simulink model "line_fit"  (Simulink 8.4)
settings: Solver=FixedStepDiscrete  SolverMode=SingleTasking  StartTime=0.0  StopTime=inf  RelTol=1e-3
model workspace (MATLAB code in the model file):
  | FracPeriod=0.5; % fraction of period of sinusoid that we will match
  | N=56; %Total number points for estimate
  | Npoly=2; % Order of polynomial to use in fitting
  | Duration = 2; % Total length of observation window
  | Ts = Duration / N; % Sample interval
undefined symbols (not defined in the file): NN
libraries: dspstat3 x3, dspsrcs4 x2, simulink x2, dsppolyfun x1, dspsnks4 x1
CloseFcn:
  | clear FixPtSimRanges;
settings Model: DataTypeOverride=Double  MinMaxOverflowLogging=MinMaxAndOverflow  Creator=Dick Benson  LastModifiedBy=Dick  ExtModeAutoUpdateStatusClock=off
settings DataIOCC: SaveOutput=off  SignalLogging=off  SaveTime=off
settings OptimizationCC: InlineParams=on  InitFltsAndDblsToZero=on
settings DebuggingCC: SignalResolutionControl=TryResolveAllWithWarning  SolverPrmCheckMsg=none
settings HardwareCC: ProdHWDeviceType=ASIC/FPGA  TargetLongLongMode=on  TargetEndianess=LittleEndian  TargetHWDeviceType=MATLAB Host  ProdEqTarget=off
settings SFSimCC: SimParseCustomCode=off
settings RTWCC: GenerateReport=on  LaunchReport=on
settings GRTTargetCC: TargetFcnLib=ansi_tfl_tmw_new.mat

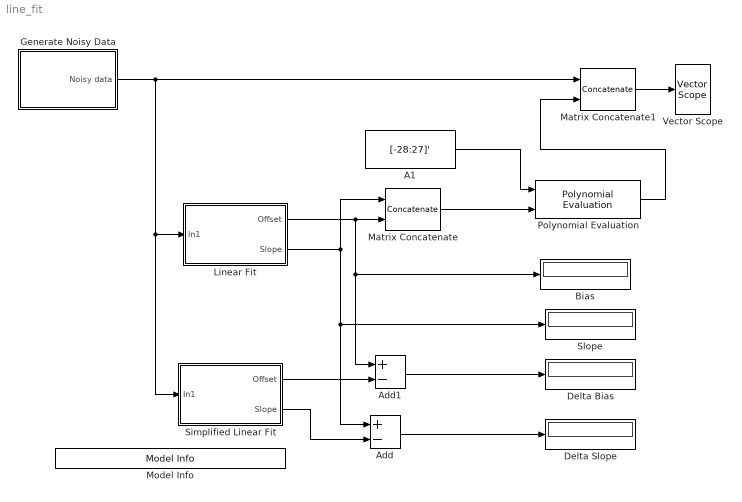
== system line_fit ==
  A1 : Constant  Value=[-28:27]'  VectorParams1D=off  OutDataTypeStr=double
  Add : Sum  Inputs=+-
  Add1 : Sum  Inputs=+-
  Bias : Display
  Delta Bias : Display
  Delta Slope : Display
  Generate Noisy Data : Subsystem
  Linear Fit : Subsystem
  Matrix Concatenate : Concatenate  Mode=Multidimensional array
  Matrix Concatenate1 : Concatenate  Mode=Multidimensional array  ConcatenateDimension=2
  Model Info : simulink/Model-Wide Utilities/Model Info  Frame=on  DisplayStringWithTags=Copyright 2008-2014 The MathWorks, Inc.  HorizontalTextAlignment=Center  LeftAlignmentValue=0.5  SourceBlockDiagram=line_fit  TagMaxNumber=20
  Polynomial Evaluation : dsppolyfun/Polynomial Evaluation  useConstCoeffs=off  constCoeffs=[5 4 3 2 1]
  Simplified Linear Fit : Subsystem
  Slope : Display
  Vector Scope : dspsnks4/Vector Scope  ScopeProperties=on  Domain=Time  HorizSpan=1  DisplayProperties=off  AxisGrid=on  Memory=off  FrameNumber=on  AxisLegend=on  AxisZoom=off  OpenScopeAtSimStart=on  OpenScopeImmediately=off  FigPos="[50   200  560   400]"  AxisProperties=off  XUnits=Hertz  XRange=[0...Fs/2]  InheritXIncr=on  XIncr=1  XLabel=Time  XLimit=Auto  XMin=0  XMax=1  XStart=0  YUnits=dB  YLabel=Amplitude  LineProperties=off  LineStyles=None  LineMarkers=.|None  LineColors=k|r  XAxisParamsVer=6.9
      settings: YMin=-5  YMax=5
  wires:
  Generate Noisy Data/1(Noisy data) -> Matrix Concatenate1/1, Linear Fit/1(In1), Simplified Linear Fit/1(In1)
  Linear Fit/1(Offset) -> Matrix Concatenate/2, Bias/1, Add1/1
  Matrix Concatenate/1 -> Polynomial Evaluation/2
  A1/1 -> Polynomial Evaluation/1
  Polynomial Evaluation/1 -> Matrix Concatenate1/2
  Linear Fit/2(Slope) -> Matrix Concatenate/1, Add/1, Slope/1
  Matrix Concatenate1/1 -> Vector Scope/1
  Simplified Linear Fit/2(Slope) -> Add/2
  Simplified Linear Fit/1(Offset) -> Add1/2
  Add/1 -> Delta Slope/1
  Add1/1 -> Delta Bias/1

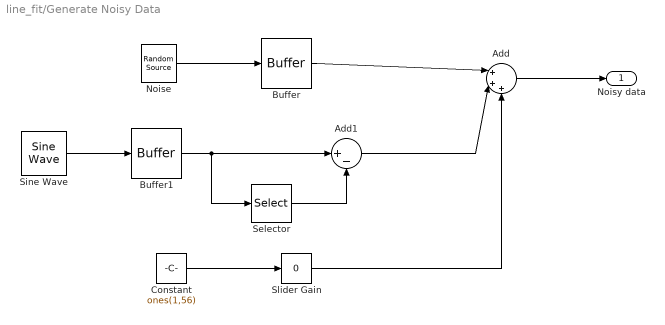
== system line_fit/Generate Noisy Data ==
  Add : Sum  Inputs=|+++
  Add1 : Sum  Inputs=|+-
  Buffer : Buffer  N=N  V=N-1  TreatMby1Signals=One channel
  Buffer1 : Buffer  N=N  V=N-1  TreatMby1Signals=One channel
  Constant : Constant  Value=ones(1,56)  SampleTime=Ts
  Noise : dspsrcs4/Random Source  SrcType=Gaussian  NormMethod=Ziggurat  CltLength=12  MinVal=0  MaxVal=1  MeanVal=0  VarVal=0.1  RepMode=Repeatable  rawSeed=1  IsInherit=off  SampMode=Discrete  SampTime=Ts  SampFrame=1  DataType=Double  OutComplex=Real
  Selector : Selector  NumberOfDimensions=2  InputPortWidth=3  IndexOptions=Index vector (dialog),Select all  Indices=1,[N+2-NN]  OutputSizes=1,NN
  Sine Wave : dspsrcs4/Sine Wave  Amplitude=1  Frequency=FracPeriod/(N*Ts)  Phase=0  SampleMode=Discrete  OutComplex=Real  CompMethod=Trigonometric fcn  TableSize=Speed  SampleTime=Ts  SamplesPerFrame=1  ResetState=Restart at time zero  dataType=double  wordLen=16  udDataType=sfix(16)  fracBitsMode=Best precision  numFracBits=15  OutDataTypeStr=double  LastOutDataTypeStr=double
  Slider Gain : simulink/Math Operations/Slider Gain  low=-2  gain=0  high=2
  Noisy data : Outport
  wires:
  Noise/1 -> Buffer/1
  Add/1 -> Noisy data/1
  Buffer1/1 -> Selector/1, Add1/1
  Buffer/1 -> Add/1
  Selector/1 -> Add1/2
  Add1/1 -> Add/2
  Sine Wave/1 -> Buffer1/1
  Constant/1 -> Slider Gain/1
  Slider Gain/1 -> Add/3

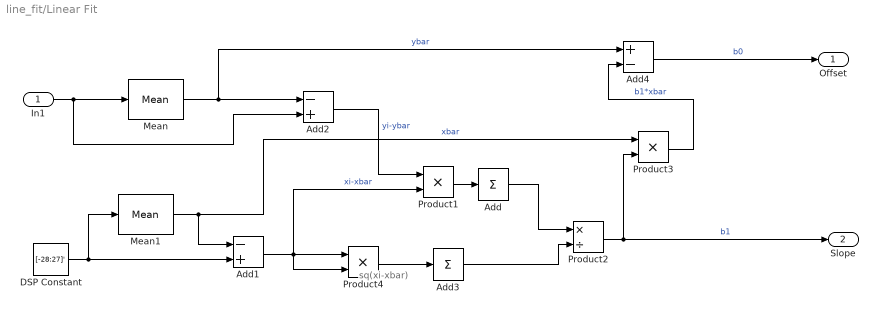
== system line_fit/Linear Fit ==
  note: sq(xi-xbar)
  In1 : Inport
  Add : Sum  Inputs=+
  Add1 : Sum  Inputs=-+
  Add2 : Sum  Inputs=-+
  Add3 : Sum  Inputs=+
  Add4 : Sum  Inputs=+-
  DSP Constant : Constant  Value=[-28:27]'  VectorParams1D=off  FramePeriod=N*Ts
      settings: SamplingMode=Frame based
  Mean : dspstat3/Mean  run=off  reset_popup=None  InputProcessing=Columns as channels (frame based)  directionMode=Each column  dimension=1  treatSBRowAsCol=on  roiEnable=off  roiType=Rectangles  roiPortion=Entire ROI  roiOutput=Individual statistics for each ROI  roiFlag=off  outputDataTypeStr=Inherit: Same as accumulator  outputLastDataTypeStr=Inherit: Same as accumulator  outputMin=[]  outputMax=[]  roundingMode=Floor  overflowMode=off
  Mean1 : dspstat3/Mean  run=off  reset_popup=None  InputProcessing=Columns as channels (frame based)  directionMode=Each column  dimension=1  treatSBRowAsCol=on  roiEnable=off  roiType=Rectangles  roiPortion=Entire ROI  roiOutput=Individual statistics for each ROI  roiFlag=off  outputDataTypeStr=Inherit: Same as accumulator  outputLastDataTypeStr=Inherit: Same as accumulator  outputMin=[]  outputMax=[]  roundingMode=Floor  overflowMode=off
  Product1 : Product  RndMeth=Zero
  Product2 : Product  Inputs=*/  RndMeth=Zero
  Product3 : Product  Inputs=**  RndMeth=Zero
  Product4 : Product  RndMeth=Zero
  Offset : Outport
  Slope : Outport  Port=2
  wires:
  DSP Constant/1 -> Mean1/1, Add1/2
  Mean1/1 -> Add1/1, Product3/1  "xbar"
  Mean/1 -> Add2/1, Add4/1  "ybar"
  Add2/1 -> Product1/1  "yi-ybar"
  Product1/1 -> Add/1
  Add/1 -> Product2/1
  Product2/1 -> Product3/2, Slope/1  "b1"
  Add3/1 -> Product2/2
  Product3/1 -> Add4/2  "b1*xbar"
  Add1/1 -> Product4/1, Product4/2, Product1/2  "xi-xbar"
  Product4/1 -> Add3/1
  In1/1 -> Mean/1, Add2/2
  Add4/1 -> Offset/1  "b0"

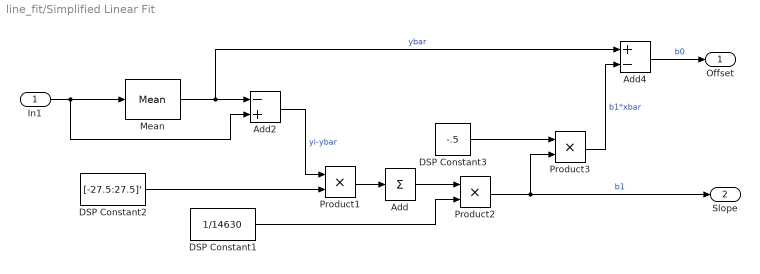
== system line_fit/Simplified Linear Fit ==
  In1 : Inport
  Add : Sum  Inputs=+
  Add2 : Sum  Inputs=-+
  Add4 : Sum  Inputs=+-
  DSP Constant1 : Constant  Value=1/14630  VectorParams1D=off  FramePeriod=N*Ts
      settings: SamplingMode=Frame based
  DSP Constant2 : Constant  Value=[-27.5:27.5]'  VectorParams1D=off  FramePeriod=N*Ts
      settings: SamplingMode=Frame based
  DSP Constant3 : Constant  Value=-.5  VectorParams1D=off  FramePeriod=N*Ts
      settings: SamplingMode=Frame based
  Mean : dspstat3/Mean  run=off  reset_popup=None  InputProcessing=Columns as channels (frame based)  directionMode=Each column  dimension=1  treatSBRowAsCol=on  roiEnable=off  roiType=Rectangles  roiPortion=Entire ROI  roiOutput=Individual statistics for each ROI  roiFlag=off  outputDataTypeStr=Inherit: Same as accumulator  outputLastDataTypeStr=Inherit: Same as accumulator  outputMin=[]  outputMax=[]  roundingMode=Floor  overflowMode=off
  Product1 : Product  RndMeth=Zero
  Product2 : Product  Inputs=**  RndMeth=Zero
  Product3 : Product  Inputs=**  RndMeth=Zero
  Offset : Outport
  Slope : Outport  Port=2
  wires:
  Add4/1 -> Offset/1  "b0"
  In1/1 -> Add2/2, Mean/1
  Product3/1 -> Add4/2  "b1*xbar"
  Product2/1 -> Slope/1, Product3/2  "b1"
  Add/1 -> Product2/1
  Product1/1 -> Add/1
  Add2/1 -> Product1/1  "yi-ybar"
  Mean/1 -> Add4/1, Add2/1  "ybar"
  DSP Constant1/1 -> Product2/2
  DSP Constant2/1 -> Product1/2
  DSP Constant3/1 -> Product3/1
